simulink model "Circuito"  (R2023b)
settings: Solver=VariableStepAuto  StartTime=0.0  StopTime=10.0  RelTol=1e-3
libraries: batteryecm_lib x10, fl_lib x1
settings Model: Creator=iangr  LastModifiedBy=iangr

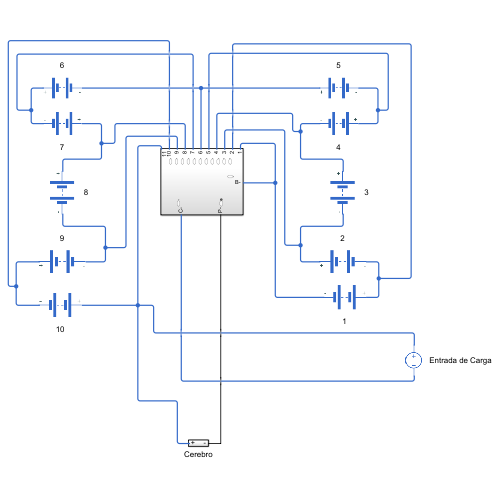
[thumbnail: Simulink's stored preview of the top-level diagram]
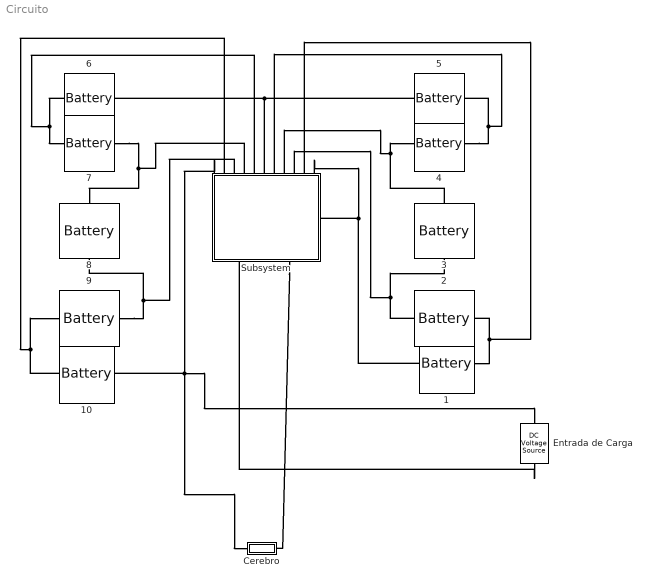
== system Circuito ==
  {1..10} (10 alike) : batteryecm_lib/Battery  Vnom=12 V  prm_dir=simscape.enum.battery.prm_dir.disabled  R1_dis=2 Ohm  R1_ch=2 Ohm  R1=2 Ohm  prm_AH=simscape.enum.battery.prm_AH.infinite  AH=50 A*hr  V1=11.5 V  AH1=25 A*hr  prm_R2=simscape.enum.battery.prm_R2.disabled  R2=2000 Ohm  Tmeas=298.15 K  charge_measurement_port=simscape.enum.battery.enable.no  prm_dyn=simscape.enum.battery.prm_dyn.off  Rp1=0.005 Ohm  tau1=30 s  Rp2=0.005 Ohm  tau2=30 s  Rp3=0.005 Ohm  tau3=30 s  Rp4=0.005 Ohm  tau4=30 s  Rp5=0.005 Ohm  tau5=30 s  prm_fade=simscape.enum.battery.prm_fade.disabled  N_fade=100  AH_fade=45 A*hr  R1_fade=2.02 Ohm  R1_ch_fade=2.02 Ohm  V1_fade=10.35 V  prm_age=simscape.enum.battery.prm_age.disabled  prm_age_OCV=simscape.enum.battery.prm_age_OCV.OCV  OCV_age=0.9  SOC_age=60  Tmeas_age=298.15 K  delta_time_age_vec=[0] d  temperature_age_vec=[273] K  OCV_scaling_age=2.2134e6  OCV_offset_age=1.632e6  temp_exp_age=0.515833569 V  t_exp_age=0.75  Vnom_T2=12 V  R1_T2=2.2 Ohm  R1_T2_dis=2.2 Ohm  R1_T2_ch=2.2 Ohm  V1_T2=11.4 V  R2_T2=2200 Ohm  Rp1_T2=0.005 Ohm  tau1_T2=30 s  Rp2_T2=0.005 Ohm  tau2_T2=30 s  Rp3_T2=0.005 Ohm  tau3_T2=30 s  Rp4_T2=0.005 Ohm  tau4_T2=30 s  Rp5_T2=0.005 Ohm  tau5_T2=30 s  Tmeas2=273.15 K  thermal_port=simscape.enum.thermaleffects.omit  thermal_mass=30000 J/K  i_specify=off  i_priority=None  i=0 A  i_nominal_specify=off  i_nominal_unit=A  i_nominal_value=1  v_specify=off  v_priority=None  v=0 V  v_nominal_specify=off  v_nominal_unit=V  v_nominal_value=1  charge_specify=off  charge_priority=High  charge=50 A*hr  charge_nominal_specify=off  charge_nominal_unit=A*hr  charge_nominal_value=1  num_cycles_specify=off  num_cycles_priority=High  num_cycles=0  num_cycles_nominal_specify=off  num_cycles_nominal_unit=1  num_cycles_nominal_value=1  temperature_specify=off  temperature_priority=High  temperature=298.15 K  temperature_nominal_specify=off  temperature_nominal_unit=K  temperature_nominal_value=1
      settings: LibrarySourceBlock=batt_lib/Cells/Battery
  Cerebro : Subsystem
  Entrada de Carga : fl_lib/Electrical/Electrical Sources/DC Voltage Source  v0=1 V
  Subsystem : Subsystem
      settings: PortSchema="{\"entries\":[{\"content\":{\"sides\":[{\"content\":{},\"type\":\"ConnectorPlacement.EquallySpacedRectSide\",\"uuid\":\"934cfeca-4efb-4867-8bd4-6afe9812654d\"},{\"content\":{\"connectorIds\":[\"RConn1\"],\"side\":\"RIGHT\"},\"type\":\"ConnectorPlacement.EquallySpacedRectSide\",\"uuid\":\"26a01779-e8e3-434e-8f21-746ce15bae26\"},{\"content\":{\"connectorIds\":[\"LConn1\",\"LConn2\",\"LConn3\",\"LConn4\",\"LConn5\",\"LConn6\",\"LConn7\",\"LConn8\",\"LConn9\",\"LConn10\",\"LConn11\"],\"side\":\"TOP\"},\"type\":\"ConnectorPlacement.EquallySpacedRectSide\",\"uuid\":\"ad3432f9-84ae-4087-a792-97c0aded843e\"},{\"content\":{\"connectorIds\":[\"RConn2\",\"RConn3\"],\"side\":\"BOTTOM\"},\"type\":\"ConnectorPlacement.EquallySpacedRectSide\",\"uuid\":\"b3867472-bb10-4cd6-9830-fe71c84d1610\"}]},\"type\":\"ConnectorPlacement.EquallySpacedConnector\",\"uuid\":\"408ff22a-25be-4301-8698-0ac970ce298c\"}],\"packageUris\":[\"http://schema.mathworks.com/mf0/Connector/R2020b\"],\"version\":\"1.0\"}"
  connections:
  1/LConn1 -- Subsystem/LConn10 -- 2/RConn1
  4/LConn1 -- Subsystem/LConn7 -- 5/RConn1
  3/LConn1 -- Subsystem/LConn8 -- 4/RConn1
  Entrada de Carga/RConn1 -- Subsystem/RConn2
  Subsystem/RConn3 -- Cerebro/RConn1
  1/RConn1 -- Subsystem/LConn11 -- Subsystem/RConn1
  2/LConn1 -- Subsystem/LConn9 -- 3/RConn1
  Subsystem/LConn1 -- 10/LConn1 -- Cerebro/LConn1 -- Entrada de Carga/LConn1
  10/RConn1 -- Subsystem/LConn2 -- 9/LConn1
  9/RConn1 -- Subsystem/LConn3 -- 8/RConn1
  5/LConn1 -- 6/RConn1 -- Subsystem/LConn6
  6/LConn1 -- Subsystem/LConn5 -- 7/RConn1
  7/LConn1 -- Subsystem/LConn4 -- 8/LConn1

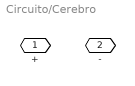
== system Circuito/Cerebro ==
  + : PMIOPort  Side=Left
  - : PMIOPort  Port=2  Side=Right

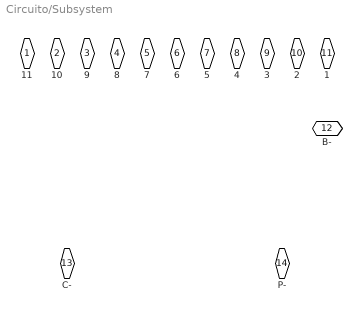
== system Circuito/Subsystem ==
  11 : PMIOPort  Side=Left
  10 : PMIOPort  Port=2  Side=Left
  9 : PMIOPort  Port=3  Side=Left
  8 : PMIOPort  Port=4  Side=Left
  7 : PMIOPort  Port=5  Side=Left
  6 : PMIOPort  Port=6  Side=Left
  5 : PMIOPort  Port=7  Side=Left
  4 : PMIOPort  Port=8  Side=Left
  3 : PMIOPort  Port=9  Side=Left
  2 : PMIOPort  Port=10  Side=Left
  1 : PMIOPort  Port=11  Side=Left
  B- : PMIOPort  Port=12  Side=Right
  C- : PMIOPort  Port=13  Side=Right
  P- : PMIOPort  Port=14  Side=Right
